simulink model "Assem1"  (R2015b)
settings: Solver=VariableStepAuto  StartTime=0.0  StopTime=10.0  RelTol=1e-3
undefined symbols (not defined in the file): Assem1, base, bearing, RootPart
libraries: mblibv1 x32
settings Model: Creator=kedar  LastModifiedBy=kedar
settings SimMechanicsCC: VisOnUpdateDiagram=on  VisDuringSimulation=on

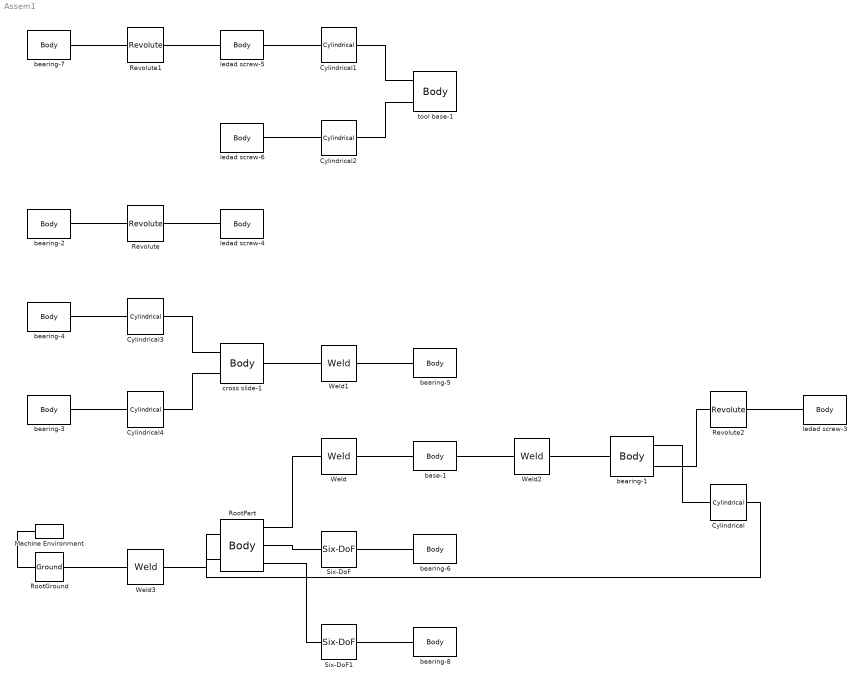
== system Assem1 ==
  Cylindrical : mblibv1/Joints/Cylindrical  LConnTagsString=__newl0  RConnTagsString=__newr0  UpdateFromCAD=on  PMImportedID=:-:Assem1/RootPart  NumSAPorts=0  CutJoint=off  MarkAsCut=off  Primitives=prismatic  PrimitiveProps=P1$WORLD$[-1,0,0]$prismatic#R1$WORLD$[1,0,0]$revolute  DialogClass=JointBlock  P1Axis=[-1,0,0]  R1Axis=[1,0,0]
  Cylindrical1 : mblibv1/Joints/Cylindrical  LConnTagsString=__newl0  RConnTagsString=__newr0  UpdateFromCAD=on  PMImportedID=ledad screw-5:-:tool base-1  NumSAPorts=0  CutJoint=off  MarkAsCut=off  Primitives=prismatic  PrimitiveProps=P1$WORLD$[0,0,-1]$prismatic#R1$WORLD$[0,0,-1]$revolute  DialogClass=JointBlock  P1Axis=[0,0,-1]  R1Axis=[0,0,-1]
  Cylindrical2 : mblibv1/Joints/Cylindrical  LConnTagsString=__newl0  RConnTagsString=__newr0  UpdateFromCAD=on  PMImportedID=ledad screw-6:-:tool base-1  NumSAPorts=0  CutJoint=off  MarkAsCut=off  Primitives=prismatic  PrimitiveProps=P1$WORLD$[0,0,-1]$prismatic#R1$WORLD$[0,0,1]$revolute  DialogClass=JointBlock  P1Axis=[0,0,-1]  R1Axis=[0,0,1]
  Cylindrical3 : mblibv1/Joints/Cylindrical  LConnTagsString=__newl0  RConnTagsString=__newr0  UpdateFromCAD=on  PMImportedID=bearing-4:-:cross slide-1  NumSAPorts=0  CutJoint=off  MarkAsCut=off  Primitives=prismatic  PrimitiveProps=P1$WORLD$[1,0,0]$prismatic#R1$WORLD$[-1,0,0]$revolute  DialogClass=JointBlock  P1Axis=[1,0,0]  R1Axis=[-1,0,0]
  Cylindrical4 : mblibv1/Joints/Cylindrical  LConnTagsString=__newl0  RConnTagsString=__newr0  UpdateFromCAD=on  PMImportedID=bearing-3:-:cross slide-1  NumSAPorts=0  CutJoint=off  MarkAsCut=off  Primitives=prismatic  PrimitiveProps=P1$WORLD$[1,0,0]$prismatic#R1$WORLD$[1,0,0]$revolute  DialogClass=JointBlock  P1Axis=[1,0,0]  R1Axis=[1,0,0]
  Machine Environment : mblibv1/Bodies/Machine Environment  PortType=env  PhysicalDomain=Mechanical  DialogTemplateClass=MECH.MachineEnvironment  SyncWhenCopied=off  Gravity=[0 -9.81 0]  GravityUnits=m/s^2  GravityAsSignal=off  Dimensionality=Auto-detect  AnalysisType=Forward dynamics  LinearAssemblyTolerance=1e-3  LinearAssemblyToleranceUnits=m  AngularAssemblyTolerance=1e-3  AngularAssemblyToleranceUnits=rad  ConstraintSolverType=Stabilizing  ConstraintRelTolerance=1e-4  ConstraintAbsTolerance=1e-4  UseRobustSingularityHandling=off  RedundancyAnalysisToleranceType=Automatically select tolerance  RedundancyAnalysisTolerance=1e-14  StatePerturbationType=Fixed  PerturbationSize=1e-5  VisualizeMachine=on  BodyVisualizationType=Use model default body geometries  BodyColorSelMode=Use model default  DefaultBodyColor=[1 0 0]
  Revolute : mblibv1/Joints/Revolute  LConnTagsString=__newl0  RConnTagsString=__newr0  UpdateFromCAD=on  PMImportedID=bearing-2:-:ledad screw-4  NumSAPorts=0  CutJoint=off  MarkAsCut=off  Primitives=prismatic  PrimitiveProps=R1$WORLD$[-1,0,0]$revolute  DialogClass=JointBlock  R1Axis=[-1,0,0]
  Revolute1 : mblibv1/Joints/Revolute  LConnTagsString=__newl0  RConnTagsString=__newr0  UpdateFromCAD=on  PMImportedID=bearing-7:-:ledad screw-5  NumSAPorts=0  CutJoint=off  MarkAsCut=off  Primitives=prismatic  PrimitiveProps=R1$WORLD$[0,0,1]$revolute  DialogClass=JointBlock  R1Axis=[0,0,1]
  Revolute2 : mblibv1/Joints/Revolute  LConnTagsString=__newl0  RConnTagsString=__newr0  UpdateFromCAD=on  PMImportedID=bearing-1:-:ledad screw-3  NumSAPorts=0  CutJoint=off  MarkAsCut=off  Primitives=prismatic  PrimitiveProps=R1$WORLD$[1,0,0]$revolute  DialogClass=JointBlock  R1Axis=[1,0,0]
  RootGround : mblibv1/Bodies/Ground  UpdateFromCAD=on  PMImportedID=RootGround  LeftPortType=env  RightPortType=workingframe  PhysicalDomain=Mechanical  DialogClass=GroundBlock  CoordPosition=[0.129768,0.219718,0.334095]  CoordPositionUnits=m  StateVectorMgrId=-1  MachineId=[0 0]  ShowEnvPort=on  ParameterChecksum=[0 0 0 0]  TopologyChecksum=[0 0 0 0]
  RootPart : mblibv1/Bodies/Body  LConnTagsString=CS3|CS4  RConnTagsString=CS2|CS5|CS6  UpdateFromCAD=on  PMImportedID=Assem1/RootPart  DialogClass=MechanicalBodyBlock  Mass=0  MassUnits=kg  InertiaUnits=kg*m^2  Inertia=[0,0,0;0,0,0;0,0,0]  Shape=Cylinder  ShapeDims=[1 1]  ShapeUnits=m  ShapeUse=false  Density=1  DensityUnits=kg/m^3  DensityUse=false  GraphicsMode=MACHINE_DEFAULT  BodyColorSelMode=MACHINE_DEFAULT  BodyColor=[1;0;0]  AttachedToCS=CS1  CG=Right$CG$[0.129768 0.219718 0.334095]$WORLD$WORLD$m$[1 0 0;0 1 0;0 0 1]$3x3 Transform$rad$WORLD$false$Assem1/RootPart::CG(AUTOGEN)  WorkingFrames=Right$CS1$[0 0 0]$WORLD$WORLD$m$[1 0 0;0 1 0;0 0 1]$3x3 Transform$rad$WORLD$false$Assem1/RootPart::CS1(AUTOGEN)#Right$CS2$[0.132232 0.182641 0.333778]$WORLD$WORLD$m$[1 0 0;0 1 0;0 0 1]$3x3 Transform$rad$WORLD$true$Assem1/RootPart:-:base-1::Assem1/RootPart(AUTOGEN)#Left$CS3$[0.312232 0.212641 0.513778]$WORLD$WORLD$m$[1 0 0;0 1 0;0 0 1]$3x3 Transform$rad$WORLD$true$:-:Assem1/RootPart::Assem1/RootPart(AUTOGEN)#Left$CS4$[0.129768 0.219718 0.334095]$WORLD$WORLD$m$[1 0 0;0 1 0;0 0 1]$3x3 Transform$rad$WORLD$true$Assem1/RootPart:-:RootGround::Assem1/RootPart(AUTOGEN)#Right$CS5$[0.129768 0.219718 0.334095]$WORLD$WORLD$m$[1 0 0;0 1 0;0 0 1]$3x3 Transform$rad$WORLD$true$Assem1/RootPart:-:bearing-6::Assem1/RootPart(AUTOGEN)#Right$CS6$[0.129768 0.219718 0.334095]$WORLD$WORLD$m$[1 0 0;0 1 0;0 0 1]$3x3 Transform$rad$WORLD$true$Assem1/RootPart:-:bearing-8::Assem1/RootPart(AUTOGEN)  CGPos=[0.129768 0.219718 0.334095]  CGRot=[1 0 0;0 1 0;0 0 1]  CS0Pos=[]  CS0Rot=[]  CS1Pos=[0 0 0]  CS1Rot=[1 0 0;0 1 0;0 0 1]  CS2Pos=[0.132232 0.182641 0.333778]  CS2Rot=[1 0 0;0 1 0;0 0 1]  CS3Pos=[0.312232 0.212641 0.513778]  CS3Rot=[1 0 0;0 1 0;0 0 1]  CS4Pos=[0.129768 0.219718 0.334095]  CS4Rot=[1 0 0;0 1 0;0 0 1]  CS5Pos=[0.129768 0.219718 0.334095]  CS5Rot=[1 0 0;0 1 0;0 0 1]  CS6Pos=[0.129768 0.219718 0.334095]  CS6Rot=[1 0 0;0 1 0;0 0 1]  CS7Pos=[]  CS7Rot=[]  CS8Pos=[]  CS8Rot=[]  CS9Pos=[]  CS9Rot=[]  CS10Pos=[]  CS10Rot=[]  CS11Pos=[]  CS11Rot=[]  CS12Pos=[]  CS12Rot=[]  CS13Pos=[]  CS13Rot=[]  CS14Pos=[]  CS14Rot=[]  CS15Pos=[]  CS15Rot=[]  CS16Pos=[]  CS16Rot=[]  CS17Pos=[]  CS17Rot=[]  CS18Pos=[]  CS18Rot=[]  CS19Pos=[]  CS19Rot=[]  CS20Pos=[]  CS20Rot=[]
  Six-DoF : mblibv1/Joints/Six-DoF  LConnTagsString=__newl0  RConnTagsString=__newr0  UpdateFromCAD=on  PMImportedID=Assem1/RootPart:-:bearing-6  NumSAPorts=0  CutJoint=off  MarkAsCut=off  Primitives=prismatic_prismatic  PrimitiveProps=P1$WORLD$[1,0,0]$prismatic#P2$WORLD$[0,1,0]$prismatic#P3$WORLD$[0,0,1]$prismatic#S$WORLD$[0,0,0]$spherical  DialogClass=JointBlock  P1Axis=[1,0,0]  P2Axis=[0,1,0]  P3Axis=[0,0,1]  SAxis=[0,0,0]
  Six-DoF1 : mblibv1/Joints/Six-DoF  LConnTagsString=__newl0  RConnTagsString=__newr0  UpdateFromCAD=on  PMImportedID=Assem1/RootPart:-:bearing-8  NumSAPorts=0  CutJoint=off  MarkAsCut=off  Primitives=prismatic_prismatic  PrimitiveProps=P1$WORLD$[1,0,0]$prismatic#P2$WORLD$[0,1,0]$prismatic#P3$WORLD$[0,0,1]$prismatic#S$WORLD$[0,0,0]$spherical  DialogClass=JointBlock  P1Axis=[1,0,0]  P2Axis=[0,1,0]  P3Axis=[0,0,1]  SAxis=[0,0,0]
  Weld : mblibv1/Joints/Weld  LConnTagsString=__newl0  RConnTagsString=__newr0  UpdateFromCAD=on  PMImportedID=Assem1/RootPart:-:base-1  NumSAPorts=0  CutJoint=off  MarkAsCut=off  Primitives=weld  PrimitiveProps=W$WORLD$[0.57735,0.57735,0.57735]$weld  DialogClass=JointBlock  WAxis=[0.57735,0.57735,0.57735]
  Weld1 : mblibv1/Joints/Weld  LConnTagsString=__newl0  RConnTagsString=__newr0  UpdateFromCAD=on  PMImportedID=bearing-5:-:cross slide-1  NumSAPorts=0  CutJoint=off  MarkAsCut=off  Primitives=weld  PrimitiveProps=W$WORLD$[0.57735,0.57735,0.57735]$weld  DialogClass=JointBlock  WAxis=[0.57735,0.57735,0.57735]
  Weld2 : mblibv1/Joints/Weld  LConnTagsString=__newl0  RConnTagsString=__newr0  UpdateFromCAD=on  PMImportedID=base-1:-:bearing-1  NumSAPorts=0  CutJoint=off  MarkAsCut=off  Primitives=weld  PrimitiveProps=W$WORLD$[0.57735,0.57735,0.57735]$weld  DialogClass=JointBlock  WAxis=[0.57735,0.57735,0.57735]
  Weld3 : mblibv1/Joints/Weld  LConnTagsString=__newl0  RConnTagsString=__newr0  UpdateFromCAD=on  PMImportedID=Assem1/RootPart:-:RootGround  NumSAPorts=0  CutJoint=off  MarkAsCut=off  Primitives=weld  PrimitiveProps=W$WORLD$[0.57735,0.57735,0.57735]$weld  DialogClass=JointBlock  WAxis=[0.57735,0.57735,0.57735]
  base-1 : mblibv1/Bodies/Body  LConnTagsString=CS2  RConnTagsString=CS3  UpdateFromCAD=on  PMImportedID=base-1  DialogClass=MechanicalBodyBlock  Mass=3.2  MassUnits=kg  InertiaUnits=kg*m^2  Inertia=[0.0427733,0,0;0,0.0853333,0;0,0,0.0427733]  Shape=Cylinder  ShapeDims=[1 1]  ShapeUnits=m  ShapeUse=false  Density=1  DensityUnits=kg/m^3  DensityUse=false  GraphicsMode=GFXFILE  GraphicsFileName=Assem1 - base-1.STL  BodyColorSelMode=COLORPALETTE  BodyColor=[0.792157;0.819608;0.933333]  AttachedToCS=CS1  CG=Right$CG$[0.132232 0.182641 0.333778]$WORLD$WORLD$m$[1 0 0;0 1 0;0 0 1]$3x3 Transform$rad$WORLD$false$base-1::CG(AUTOGEN)  WorkingFrames=Right$CS1$[0.132232 0.172641 0.333778]$WORLD$WORLD$m$[1 0 0;0 1 0;0 0 1]$3x3 Transform$rad$WORLD$false$base-1::CS1(AUTOGEN)#Left$CS2$[0.132232 0.182641 0.333778]$WORLD$WORLD$m$[1 0 0;0 1 0;0 0 1]$3x3 Transform$rad$WORLD$true$Assem1/RootPart:-:base-1::base-1(AUTOGEN)#Right$CS3$[0.332232 0.192641 0.533778]$WORLD$WORLD$m$[1 0 0;0 1 0;0 0 1]$3x3 Transform$rad$WORLD$true$base-1:-:bearing-1::base-1(AUTOGEN)  CGPos=[0.132232 0.182641 0.333778]  CGRot=[1 0 0;0 1 0;0 0 1]  CS0Pos=[]  CS0Rot=[]  CS1Pos=[0.132232 0.172641 0.333778]  CS1Rot=[1 0 0;0 1 0;0 0 1]  CS2Pos=[0.132232 0.182641 0.333778]  CS2Rot=[1 0 0;0 1 0;0 0 1]  CS3Pos=[0.332232 0.192641 0.533778]  CS3Rot=[1 0 0;0 1 0;0 0 1]  CS4Pos=[]  CS4Rot=[]  CS5Pos=[]  CS5Rot=[]  CS6Pos=[]  CS6Rot=[]  CS7Pos=[]  CS7Rot=[]  CS8Pos=[]  CS8Rot=[]  CS9Pos=[]  CS9Rot=[]  CS10Pos=[]  CS10Rot=[]  CS11Pos=[]  CS11Rot=[]  CS12Pos=[]  CS12Rot=[]  CS13Pos=[]  CS13Rot=[]  CS14Pos=[]  CS14Rot=[]  CS15Pos=[]  CS15Rot=[]  CS16Pos=[]  CS16Rot=[]  CS17Pos=[]  CS17Rot=[]  CS18Pos=[]  CS18Rot=[]  CS19Pos=[]  CS19Rot=[]  CS20Pos=[]  CS20Rot=[]
  bearing-1 : mblibv1/Bodies/Body  LConnTagsString=CS3  RConnTagsString=CS2|CS4  UpdateFromCAD=on  PMImportedID=bearing-1  DialogClass=MechanicalBodyBlock  Mass=0.0240913  MassUnits=kg  InertiaUnits=kg*m^2  Inertia=[4.82084e-06,0,0;0,4.82084e-06,0;0,0,8.03559e-06]  Shape=Cylinder  ShapeDims=[1 1]  ShapeUnits=m  ShapeUse=false  Density=1  DensityUnits=kg/m^3  DensityUse=false  GraphicsMode=GFXFILE  GraphicsFileName=Assem1 - bearing-1.STL  BodyColorSelMode=COLORPALETTE  BodyColor=[0.792157;0.819608;0.933333]  AttachedToCS=CS1  CG=Right$CG$[0.322232 0.212641 0.513778]$WORLD$WORLD$m$[0 0 -1;0 -1 0;-1 0 0]$3x3 Transform$rad$WORLD$false$bearing-1::CG(AUTOGEN)  WorkingFrames=Right$CS1$[0.332232 0.212641 0.513778]$WORLD$WORLD$m$[0 0 -1;0 -1 0;-1 0 0]$3x3 Transform$rad$WORLD$false$bearing-1::CS1(AUTOGEN)#Right$CS2$[0.312232 0.212641 0.513778]$WORLD$WORLD$m$[1 0 0;0 1 0;0 0 1]$3x3 Transform$rad$WORLD$true$:-:Assem1/RootPart::bearing-1(AUTOGEN)#Left$CS3$[0.332232 0.192641 0.533778]$WORLD$WORLD$m$[1 0 0;0 1 0;0 0 1]$3x3 Transform$rad$WORLD$true$base-1:-:bearing-1::bearing-1(AUTOGEN)#Right$CS4$[0.312232 0.212641 0.513778]$WORLD$WORLD$m$[1 0 0;0 1 0;0 0 1]$3x3 Transform$rad$WORLD$true$bearing-1:-:ledad screw-3::bearing-1(AUTOGEN)  CGPos=[0.322232 0.212641 0.513778]  CGRot=[0 0 -1;0 -1 0;-1 0 0]  CS0Pos=[]  CS0Rot=[]  CS1Pos=[0.332232 0.212641 0.513778]  CS1Rot=[0 0 -1;0 -1 0;-1 0 0]  CS2Pos=[0.312232 0.212641 0.513778]  CS2Rot=[1 0 0;0 1 0;0 0 1]  CS3Pos=[0.332232 0.192641 0.533778]  CS3Rot=[1 0 0;0 1 0;0 0 1]  CS4Pos=[0.312232 0.212641 0.513778]  CS4Rot=[1 0 0;0 1 0;0 0 1]  CS5Pos=[]  CS5Rot=[]  CS6Pos=[]  CS6Rot=[]  CS7Pos=[]  CS7Rot=[]  CS8Pos=[]  CS8Rot=[]  CS9Pos=[]  CS9Rot=[]  CS10Pos=[]  CS10Rot=[]  CS11Pos=[]  CS11Rot=[]  CS12Pos=[]  CS12Rot=[]  CS13Pos=[]  CS13Rot=[]  CS14Pos=[]  CS14Rot=[]  CS15Pos=[]  CS15Rot=[]  CS16Pos=[]  CS16Rot=[]  CS17Pos=[]  CS17Rot=[]  CS18Pos=[]  CS18Rot=[]  CS19Pos=[]  CS19Rot=[]  CS20Pos=[]  CS20Rot=[]
  bearing-2 : mblibv1/Bodies/Body  RConnTagsString=CS2  UpdateFromCAD=on  PMImportedID=bearing-2  DialogClass=MechanicalBodyBlock  Mass=0.0240913  MassUnits=kg  InertiaUnits=kg*m^2  Inertia=[4.82084e-06,0,0;0,4.82084e-06,0;0,0,8.03559e-06]  Shape=Cylinder  ShapeDims=[1 1]  ShapeUnits=m  ShapeUse=false  Density=1  DensityUnits=kg/m^3  DensityUse=false  GraphicsMode=GFXFILE  GraphicsFileName=Assem1 - bearing-2.STL  BodyColorSelMode=COLORPALETTE  BodyColor=[0.792157;0.819608;0.933333]  AttachedToCS=CS1  CG=Right$CG$[0.322232 0.212641 0.153778]$WORLD$WORLD$m$[0 0 1;0 -1 0;1 0 0]$3x3 Transform$rad$WORLD$false$bearing-2::CG(AUTOGEN)  WorkingFrames=Right$CS1$[0.312232 0.212641 0.153778]$WORLD$WORLD$m$[0 0 1;0 -1 0;1 0 0]$3x3 Transform$rad$WORLD$false$bearing-2::CS1(AUTOGEN)#Right$CS2$[0.332232 0.212641 0.153778]$WORLD$WORLD$m$[1 0 0;0 1 0;0 0 1]$3x3 Transform$rad$WORLD$true$bearing-2:-:ledad screw-4::bearing-2(AUTOGEN)  CGPos=[0.322232 0.212641 0.153778]  CGRot=[0 0 1;0 -1 0;1 0 0]  CS0Pos=[]  CS0Rot=[]  CS1Pos=[0.312232 0.212641 0.153778]  CS1Rot=[0 0 1;0 -1 0;1 0 0]  CS2Pos=[0.332232 0.212641 0.153778]  CS2Rot=[1 0 0;0 1 0;0 0 1]  CS3Pos=[]  CS3Rot=[]  CS4Pos=[]  CS4Rot=[]  CS5Pos=[]  CS5Rot=[]  CS6Pos=[]  CS6Rot=[]  CS7Pos=[]  CS7Rot=[]  CS8Pos=[]  CS8Rot=[]  CS9Pos=[]  CS9Rot=[]  CS10Pos=[]  CS10Rot=[]  CS11Pos=[]  CS11Rot=[]  CS12Pos=[]  CS12Rot=[]  CS13Pos=[]  CS13Rot=[]  CS14Pos=[]  CS14Rot=[]  CS15Pos=[]  CS15Rot=[]  CS16Pos=[]  CS16Rot=[]  CS17Pos=[]  CS17Rot=[]  CS18Pos=[]  CS18Rot=[]  CS19Pos=[]  CS19Rot=[]  CS20Pos=[]  CS20Rot=[]
  bearing-3 : mblibv1/Bodies/Body  RConnTagsString=CS2  UpdateFromCAD=on  PMImportedID=bearing-3  DialogClass=MechanicalBodyBlock  Mass=0.0240913  MassUnits=kg  InertiaUnits=kg*m^2  Inertia=[4.82084e-06,0,0;0,4.82084e-06,0;0,0,8.03559e-06]  Shape=Cylinder  ShapeDims=[1 1]  ShapeUnits=m  ShapeUse=false  Density=1  DensityUnits=kg/m^3  DensityUse=false  GraphicsMode=GFXFILE  GraphicsFileName=Assem1 - bearing-3.STL  BodyColorSelMode=COLORPALETTE  BodyColor=[0.792157;0.819608;0.933333]  AttachedToCS=CS1  CG=Right$CG$[-0.0577677 0.212641 0.513778]$WORLD$WORLD$m$[0 0 -1;0 -1 0;-1 0 0]$3x3 Transform$rad$WORLD$false$bearing-3::CG(AUTOGEN)  WorkingFrames=Right$CS1$[-0.0477677 0.212641 0.513778]$WORLD$WORLD$m$[0 0 -1;0 -1 0;-1 0 0]$3x3 Transform$rad$WORLD$false$bearing-3::CS1(AUTOGEN)#Right$CS2$[-0.0677677 0.212641 0.513778]$WORLD$WORLD$m$[1 0 0;0 1 0;0 0 1]$3x3 Transform$rad$WORLD$true$bearing-3:-:cross slide-1::bearing-3(AUTOGEN)  CGPos=[-0.0577677 0.212641 0.513778]  CGRot=[0 0 -1;0 -1 0;-1 0 0]  CS0Pos=[]  CS0Rot=[]  CS1Pos=[-0.0477677 0.212641 0.513778]  CS1Rot=[0 0 -1;0 -1 0;-1 0 0]  CS2Pos=[-0.0677677 0.212641 0.513778]  CS2Rot=[1 0 0;0 1 0;0 0 1]  CS3Pos=[]  CS3Rot=[]  CS4Pos=[]  CS4Rot=[]  CS5Pos=[]  CS5Rot=[]  CS6Pos=[]  CS6Rot=[]  CS7Pos=[]  CS7Rot=[]  CS8Pos=[]  CS8Rot=[]  CS9Pos=[]  CS9Rot=[]  CS10Pos=[]  CS10Rot=[]  CS11Pos=[]  CS11Rot=[]  CS12Pos=[]  CS12Rot=[]  CS13Pos=[]  CS13Rot=[]  CS14Pos=[]  CS14Rot=[]  CS15Pos=[]  CS15Rot=[]  CS16Pos=[]  CS16Rot=[]  CS17Pos=[]  CS17Rot=[]  CS18Pos=[]  CS18Rot=[]  CS19Pos=[]  CS19Rot=[]  CS20Pos=[]  CS20Rot=[]
  bearing-4 : mblibv1/Bodies/Body  RConnTagsString=CS2  UpdateFromCAD=on  PMImportedID=bearing-4  DialogClass=MechanicalBodyBlock  Mass=0.0240913  MassUnits=kg  InertiaUnits=kg*m^2  Inertia=[4.82084e-06,0,0;0,4.82084e-06,0;0,0,8.03559e-06]  Shape=Cylinder  ShapeDims=[1 1]  ShapeUnits=m  ShapeUse=false  Density=1  DensityUnits=kg/m^3  DensityUse=false  GraphicsMode=GFXFILE  GraphicsFileName=Assem1 - bearing-4.STL  BodyColorSelMode=COLORPALETTE  BodyColor=[0.792157;0.819608;0.933333]  AttachedToCS=CS1  CG=Right$CG$[-0.0577677 0.212641 0.153778]$WORLD$WORLD$m$[0 0 1;0 -1 0;1 0 0]$3x3 Transform$rad$WORLD$false$bearing-4::CG(AUTOGEN)  WorkingFrames=Right$CS1$[-0.0677677 0.212641 0.153778]$WORLD$WORLD$m$[0 0 1;0 -1 0;1 0 0]$3x3 Transform$rad$WORLD$false$bearing-4::CS1(AUTOGEN)#Right$CS2$[-0.0477677 0.212641 0.153778]$WORLD$WORLD$m$[1 0 0;0 1 0;0 0 1]$3x3 Transform$rad$WORLD$true$bearing-4:-:cross slide-1::bearing-4(AUTOGEN)  CGPos=[-0.0577677 0.212641 0.153778]  CGRot=[0 0 1;0 -1 0;1 0 0]  CS0Pos=[]  CS0Rot=[]  CS1Pos=[-0.0677677 0.212641 0.153778]  CS1Rot=[0 0 1;0 -1 0;1 0 0]  CS2Pos=[-0.0477677 0.212641 0.153778]  CS2Rot=[1 0 0;0 1 0;0 0 1]  CS3Pos=[]  CS3Rot=[]  CS4Pos=[]  CS4Rot=[]  CS5Pos=[]  CS5Rot=[]  CS6Pos=[]  CS6Rot=[]  CS7Pos=[]  CS7Rot=[]  CS8Pos=[]  CS8Rot=[]  CS9Pos=[]  CS9Rot=[]  CS10Pos=[]  CS10Rot=[]  CS11Pos=[]  CS11Rot=[]  CS12Pos=[]  CS12Rot=[]  CS13Pos=[]  CS13Rot=[]  CS14Pos=[]  CS14Rot=[]  CS15Pos=[]  CS15Rot=[]  CS16Pos=[]  CS16Rot=[]  CS17Pos=[]  CS17Rot=[]  CS18Pos=[]  CS18Rot=[]  CS19Pos=[]  CS19Rot=[]  CS20Pos=[]  CS20Rot=[]
  bearing-5 : mblibv1/Bodies/Body  LConnTagsString=CS2  UpdateFromCAD=on  PMImportedID=bearing-5  DialogClass=MechanicalBodyBlock  Mass=0.0240913  MassUnits=kg  InertiaUnits=kg*m^2  Inertia=[4.82084e-06,0,0;0,4.82084e-06,0;0,0,8.03559e-06]  Shape=Cylinder  ShapeDims=[1 1]  ShapeUnits=m  ShapeUse=false  Density=1  DensityUnits=kg/m^3  DensityUse=false  GraphicsMode=GFXFILE  GraphicsFileName=Assem1 - bearing-5.STL  BodyColorSelMode=COLORPALETTE  BodyColor=[0.792157;0.819608;0.933333]  AttachedToCS=CS1  CG=Right$CG$[0.236818 0.272641 0.523778]$WORLD$WORLD$m$[1 0 0;0 1 0;0 0 1]$3x3 Transform$rad$WORLD$false$bearing-5::CG(AUTOGEN)  WorkingFrames=Right$CS1$[0.236818 0.272641 0.513778]$WORLD$WORLD$m$[1 0 0;0 1 0;0 0 1]$3x3 Transform$rad$WORLD$false$bearing-5::CS1(AUTOGEN)#Left$CS2$[0.256818 0.232641 0.133778]$WORLD$WORLD$m$[1 0 0;0 1 0;0 0 1]$3x3 Transform$rad$WORLD$true$bearing-5:-:cross slide-1::bearing-5(AUTOGEN)  CGPos=[0.236818 0.272641 0.523778]  CGRot=[1 0 0;0 1 0;0 0 1]  CS0Pos=[]  CS0Rot=[]  CS1Pos=[0.236818 0.272641 0.513778]  CS1Rot=[1 0 0;0 1 0;0 0 1]  CS2Pos=[0.256818 0.232641 0.133778]  CS2Rot=[1 0 0;0 1 0;0 0 1]  CS3Pos=[]  CS3Rot=[]  CS4Pos=[]  CS4Rot=[]  CS5Pos=[]  CS5Rot=[]  CS6Pos=[]  CS6Rot=[]  CS7Pos=[]  CS7Rot=[]  CS8Pos=[]  CS8Rot=[]  CS9Pos=[]  CS9Rot=[]  CS10Pos=[]  CS10Rot=[]  CS11Pos=[]  CS11Rot=[]  CS12Pos=[]  CS12Rot=[]  CS13Pos=[]  CS13Rot=[]  CS14Pos=[]  CS14Rot=[]  CS15Pos=[]  CS15Rot=[]  CS16Pos=[]  CS16Rot=[]  CS17Pos=[]  CS17Rot=[]  CS18Pos=[]  CS18Rot=[]  CS19Pos=[]  CS19Rot=[]  CS20Pos=[]  CS20Rot=[]
  bearing-6 : mblibv1/Bodies/Body  LConnTagsString=CS2  UpdateFromCAD=on  PMImportedID=bearing-6  DialogClass=MechanicalBodyBlock  Mass=0.0240913  MassUnits=kg  InertiaUnits=kg*m^2  Inertia=[4.82084e-06,0,0;0,4.82084e-06,0;0,0,8.03559e-06]  Shape=Cylinder  ShapeDims=[1 1]  ShapeUnits=m  ShapeUse=false  Density=1  DensityUnits=kg/m^3  DensityUse=false  GraphicsMode=GFXFILE  GraphicsFileName=Assem1 - bearing-6.STL  BodyColorSelMode=COLORPALETTE  BodyColor=[0.792157;0.819608;0.933333]  AttachedToCS=CS1  CG=Right$CG$[0.236818 0.272641 0.143778]$WORLD$WORLD$m$[1 0 0;0 1 0;0 0 1]$3x3 Transform$rad$WORLD$false$bearing-6::CG(AUTOGEN)  WorkingFrames=Right$CS1$[0.236818 0.272641 0.133778]$WORLD$WORLD$m$[1 0 0;0 1 0;0 0 1]$3x3 Transform$rad$WORLD$false$bearing-6::CS1(AUTOGEN)#Left$CS2$[0.236818 0.272641 0.143778]$WORLD$WORLD$m$[1 0 0;0 1 0;0 0 1]$3x3 Transform$rad$WORLD$true$Assem1/RootPart:-:bearing-6::bearing-6(AUTOGEN)  CGPos=[0.236818 0.272641 0.143778]  CGRot=[1 0 0;0 1 0;0 0 1]  CS0Pos=[]  CS0Rot=[]  CS1Pos=[0.236818 0.272641 0.133778]  CS1Rot=[1 0 0;0 1 0;0 0 1]  CS2Pos=[0.236818 0.272641 0.143778]  CS2Rot=[1 0 0;0 1 0;0 0 1]  CS3Pos=[]  CS3Rot=[]  CS4Pos=[]  CS4Rot=[]  CS5Pos=[]  CS5Rot=[]  CS6Pos=[]  CS6Rot=[]  CS7Pos=[]  CS7Rot=[]  CS8Pos=[]  CS8Rot=[]  CS9Pos=[]  CS9Rot=[]  CS10Pos=[]  CS10Rot=[]  CS11Pos=[]  CS11Rot=[]  CS12Pos=[]  CS12Rot=[]  CS13Pos=[]  CS13Rot=[]  CS14Pos=[]  CS14Rot=[]  CS15Pos=[]  CS15Rot=[]  CS16Pos=[]  CS16Rot=[]  CS17Pos=[]  CS17Rot=[]  CS18Pos=[]  CS18Rot=[]  CS19Pos=[]  CS19Rot=[]  CS20Pos=[]  CS20Rot=[]
  bearing-7 : mblibv1/Bodies/Body  RConnTagsString=CS2  UpdateFromCAD=on  PMImportedID=bearing-7  DialogClass=MechanicalBodyBlock  Mass=0.0240913  MassUnits=kg  InertiaUnits=kg*m^2  Inertia=[4.82084e-06,0,0;0,4.82084e-06,0;0,0,8.03559e-06]  Shape=Cylinder  ShapeDims=[1 1]  ShapeUnits=m  ShapeUse=false  Density=1  DensityUnits=kg/m^3  DensityUse=false  GraphicsMode=GFXFILE  GraphicsFileName=Assem1 - bearing-7.STL  BodyColorSelMode=COLORPALETTE  BodyColor=[0.792157;0.819608;0.933333]  AttachedToCS=CS1  CG=Right$CG$[0.0268176 0.272641 0.523778]$WORLD$WORLD$m$[-1 0 0;0 1 0;0 0 -1]$3x3 Transform$rad$WORLD$false$bearing-7::CG(AUTOGEN)  WorkingFrames=Right$CS1$[0.0268176 0.272641 0.533778]$WORLD$WORLD$m$[-1 0 0;0 1 0;0 0 -1]$3x3 Transform$rad$WORLD$false$bearing-7::CS1(AUTOGEN)#Right$CS2$[0.0268176 0.272641 0.513778]$WORLD$WORLD$m$[1 0 0;0 1 0;0 0 1]$3x3 Transform$rad$WORLD$true$bearing-7:-:ledad screw-5::bearing-7(AUTOGEN)  CGPos=[0.0268176 0.272641 0.523778]  CGRot=[-1 0 0;0 1 0;0 0 -1]  CS0Pos=[]  CS0Rot=[]  CS1Pos=[0.0268176 0.272641 0.533778]  CS1Rot=[-1 0 0;0 1 0;0 0 -1]  CS2Pos=[0.0268176 0.272641 0.513778]  CS2Rot=[1 0 0;0 1 0;0 0 1]  CS3Pos=[]  CS3Rot=[]  CS4Pos=[]  CS4Rot=[]  CS5Pos=[]  CS5Rot=[]  CS6Pos=[]  CS6Rot=[]  CS7Pos=[]  CS7Rot=[]  CS8Pos=[]  CS8Rot=[]  CS9Pos=[]  CS9Rot=[]  CS10Pos=[]  CS10Rot=[]  CS11Pos=[]  CS11Rot=[]  CS12Pos=[]  CS12Rot=[]  CS13Pos=[]  CS13Rot=[]  CS14Pos=[]  CS14Rot=[]  CS15Pos=[]  CS15Rot=[]  CS16Pos=[]  CS16Rot=[]  CS17Pos=[]  CS17Rot=[]  CS18Pos=[]  CS18Rot=[]  CS19Pos=[]  CS19Rot=[]  CS20Pos=[]  CS20Rot=[]
  bearing-8 : mblibv1/Bodies/Body  LConnTagsString=CS2  UpdateFromCAD=on  PMImportedID=bearing-8  DialogClass=MechanicalBodyBlock  Mass=0.0240913  MassUnits=kg  InertiaUnits=kg*m^2  Inertia=[4.82084e-06,0,0;0,4.82084e-06,0;0,0,8.03559e-06]  Shape=Cylinder  ShapeDims=[1 1]  ShapeUnits=m  ShapeUse=false  Density=1  DensityUnits=kg/m^3  DensityUse=false  GraphicsMode=GFXFILE  GraphicsFileName=Assem1 - bearing-8.STL  BodyColorSelMode=COLORPALETTE  BodyColor=[0.792157;0.819608;0.933333]  AttachedToCS=CS1  CG=Right$CG$[0.0268176 0.272641 0.143778]$WORLD$WORLD$m$[-1 0 0;0 1 0;0 0 -1]$3x3 Transform$rad$WORLD$false$bearing-8::CG(AUTOGEN)  WorkingFrames=Right$CS1$[0.0268176 0.272641 0.153778]$WORLD$WORLD$m$[-1 0 0;0 1 0;0 0 -1]$3x3 Transform$rad$WORLD$false$bearing-8::CS1(AUTOGEN)#Left$CS2$[0.0268176 0.272641 0.143778]$WORLD$WORLD$m$[1 0 0;0 1 0;0 0 1]$3x3 Transform$rad$WORLD$true$Assem1/RootPart:-:bearing-8::bearing-8(AUTOGEN)  CGPos=[0.0268176 0.272641 0.143778]  CGRot=[-1 0 0;0 1 0;0 0 -1]  CS0Pos=[]  CS0Rot=[]  CS1Pos=[0.0268176 0.272641 0.153778]  CS1Rot=[-1 0 0;0 1 0;0 0 -1]  CS2Pos=[0.0268176 0.272641 0.143778]  CS2Rot=[1 0 0;0 1 0;0 0 1]  CS3Pos=[]  CS3Rot=[]  CS4Pos=[]  CS4Rot=[]  CS5Pos=[]  CS5Rot=[]  CS6Pos=[]  CS6Rot=[]  CS7Pos=[]  CS7Rot=[]  CS8Pos=[]  CS8Rot=[]  CS9Pos=[]  CS9Rot=[]  CS10Pos=[]  CS10Rot=[]  CS11Pos=[]  CS11Rot=[]  CS12Pos=[]  CS12Rot=[]  CS13Pos=[]  CS13Rot=[]  CS14Pos=[]  CS14Rot=[]  CS15Pos=[]  CS15Rot=[]  CS16Pos=[]  CS16Rot=[]  CS17Pos=[]  CS17Rot=[]  CS18Pos=[]  CS18Rot=[]  CS19Pos=[]  CS19Rot=[]  CS20Pos=[]  CS20Rot=[]
  cross slide-1 : mblibv1/Bodies/Body  LConnTagsString=CS3|CS4  RConnTagsString=CS2  UpdateFromCAD=on  PMImportedID=cross slide-1  DialogClass=MechanicalBodyBlock  Mass=2.1543  MassUnits=kg  InertiaUnits=kg*m^2  Inertia=[0.0125155,0,0;0,0.043986,0;0,0,0.0319109]  Shape=Cylinder  ShapeDims=[1 1]  ShapeUnits=m  ShapeUse=false  Density=1  DensityUnits=kg/m^3  DensityUse=false  GraphicsMode=GFXFILE  GraphicsFileName=Assem1 - cross slide-1.STL  BodyColorSelMode=COLORPALETTE  BodyColor=[0.792157;0.819608;0.933333]  AttachedToCS=CS1  CG=Right$CG$[0.131818 0.240492 0.333778]$WORLD$WORLD$m$[0 0 1;0 -1 0;1 0 0]$3x3 Transform$rad$WORLD$false$cross slide-1::CG(AUTOGEN)  WorkingFrames=Right$CS1$[0.131818 0.252641 0.333778]$WORLD$WORLD$m$[0 0 1;0 -1 0;1 0 0]$3x3 Transform$rad$WORLD$false$cross slide-1::CS1(AUTOGEN)#Right$CS2$[0.256818 0.232641 0.133778]$WORLD$WORLD$m$[1 0 0;0 1 0;0 0 1]$3x3 Transform$rad$WORLD$true$bearing-5:-:cross slide-1::cross slide-1(AUTOGEN)#Left$CS3$[-0.0477677 0.212641 0.153778]$WORLD$WORLD$m$[1 0 0;0 1 0;0 0 1]$3x3 Transform$rad$WORLD$true$bearing-4:-:cross slide-1::cross slide-1(AUTOGEN)#Left$CS4$[-0.0677677 0.212641 0.513778]$WORLD$WORLD$m$[1 0 0;0 1 0;0 0 1]$3x3 Transform$rad$WORLD$true$bearing-3:-:cross slide-1::cross slide-1(AUTOGEN)  CGPos=[0.131818 0.240492 0.333778]  CGRot=[0 0 1;0 -1 0;1 0 0]  CS0Pos=[]  CS0Rot=[]  CS1Pos=[0.131818 0.252641 0.333778]  CS1Rot=[0 0 1;0 -1 0;1 0 0]  CS2Pos=[0.256818 0.232641 0.133778]  CS2Rot=[1 0 0;0 1 0;0 0 1]  CS3Pos=[-0.0477677 0.212641 0.153778]  CS3Rot=[1 0 0;0 1 0;0 0 1]  CS4Pos=[-0.0677677 0.212641 0.513778]  CS4Rot=[1 0 0;0 1 0;0 0 1]  CS5Pos=[]  CS5Rot=[]  CS6Pos=[]  CS6Rot=[]  CS7Pos=[]  CS7Rot=[]  CS8Pos=[]  CS8Rot=[]  CS9Pos=[]  CS9Rot=[]  CS10Pos=[]  CS10Rot=[]  CS11Pos=[]  CS11Rot=[]  CS12Pos=[]  CS12Rot=[]  CS13Pos=[]  CS13Rot=[]  CS14Pos=[]  CS14Rot=[]  CS15Pos=[]  CS15Rot=[]  CS16Pos=[]  CS16Rot=[]  CS17Pos=[]  CS17Rot=[]  CS18Pos=[]  CS18Rot=[]  CS19Pos=[]  CS19Rot=[]  CS20Pos=[]  CS20Rot=[]
  ledad screw-3 : mblibv1/Bodies/Body  LConnTagsString=CS2  UpdateFromCAD=on  PMImportedID=ledad screw-3  DialogClass=MechanicalBodyBlock  Mass=0.15708  MassUnits=kg  InertiaUnits=kg*m^2  Inertia=[0.00327642,0,0;0,0.00327642,0;0,0,7.85398e-06]  Shape=Cylinder  ShapeDims=[1 1]  ShapeUnits=m  ShapeUse=false  Density=1  DensityUnits=kg/m^3  DensityUse=false  GraphicsMode=GFXFILE  GraphicsFileName=Assem1 - ledad screw-3.STL  BodyColorSelMode=COLORPALETTE  BodyColor=[0.792157;0.819608;0.933333]  AttachedToCS=CS1  CG=Right$CG$[0.0822323 0.212641 0.513778]$WORLD$WORLD$m$[0 0 1;0 1 0;-1 0 0]$3x3 Transform$rad$WORLD$false$ledad screw-3::CG(AUTOGEN)  WorkingFrames=Right$CS1$[-0.167768 0.212641 0.513778]$WORLD$WORLD$m$[0 0 1;0 1 0;-1 0 0]$3x3 Transform$rad$WORLD$false$ledad screw-3::CS1(AUTOGEN)#Left$CS2$[0.312232 0.212641 0.513778]$WORLD$WORLD$m$[1 0 0;0 1 0;0 0 1]$3x3 Transform$rad$WORLD$true$bearing-1:-:ledad screw-3::ledad screw-3(AUTOGEN)  CGPos=[0.0822323 0.212641 0.513778]  CGRot=[0 0 1;0 1 0;-1 0 0]  CS0Pos=[]  CS0Rot=[]  CS1Pos=[-0.167768 0.212641 0.513778]  CS1Rot=[0 0 1;0 1 0;-1 0 0]  CS2Pos=[0.312232 0.212641 0.513778]  CS2Rot=[1 0 0;0 1 0;0 0 1]  CS3Pos=[]  CS3Rot=[]  CS4Pos=[]  CS4Rot=[]  CS5Pos=[]  CS5Rot=[]  CS6Pos=[]  CS6Rot=[]  CS7Pos=[]  CS7Rot=[]  CS8Pos=[]  CS8Rot=[]  CS9Pos=[]  CS9Rot=[]  CS10Pos=[]  CS10Rot=[]  CS11Pos=[]  CS11Rot=[]  CS12Pos=[]  CS12Rot=[]  CS13Pos=[]  CS13Rot=[]  CS14Pos=[]  CS14Rot=[]  CS15Pos=[]  CS15Rot=[]  CS16Pos=[]  CS16Rot=[]  CS17Pos=[]  CS17Rot=[]  CS18Pos=[]  CS18Rot=[]  CS19Pos=[]  CS19Rot=[]  CS20Pos=[]  CS20Rot=[]
  ledad screw-4 : mblibv1/Bodies/Body  LConnTagsString=CS2  UpdateFromCAD=on  PMImportedID=ledad screw-4  DialogClass=MechanicalBodyBlock  Mass=0.15708  MassUnits=kg  InertiaUnits=kg*m^2  Inertia=[0.00327642,0,0;0,0.00327642,0;0,0,7.85398e-06]  Shape=Cylinder  ShapeDims=[1 1]  ShapeUnits=m  ShapeUse=false  Density=1  DensityUnits=kg/m^3  DensityUse=false  GraphicsMode=GFXFILE  GraphicsFileName=Assem1 - ledad screw-4.STL  BodyColorSelMode=COLORPALETTE  BodyColor=[0.792157;0.819608;0.933333]  AttachedToCS=CS1  CG=Right$CG$[0.0822323 0.212641 0.153778]$WORLD$WORLD$m$[0 0 -1;0 1 0;1 0 0]$3x3 Transform$rad$WORLD$false$ledad screw-4::CG(AUTOGEN)  WorkingFrames=Right$CS1$[0.332232 0.212641 0.153778]$WORLD$WORLD$m$[0 0 -1;0 1 0;1 0 0]$3x3 Transform$rad$WORLD$false$ledad screw-4::CS1(AUTOGEN)#Left$CS2$[0.332232 0.212641 0.153778]$WORLD$WORLD$m$[1 0 0;0 1 0;0 0 1]$3x3 Transform$rad$WORLD$true$bearing-2:-:ledad screw-4::ledad screw-4(AUTOGEN)  CGPos=[0.0822323 0.212641 0.153778]  CGRot=[0 0 -1;0 1 0;1 0 0]  CS0Pos=[]  CS0Rot=[]  CS1Pos=[0.332232 0.212641 0.153778]  CS1Rot=[0 0 -1;0 1 0;1 0 0]  CS2Pos=[0.332232 0.212641 0.153778]  CS2Rot=[1 0 0;0 1 0;0 0 1]  CS3Pos=[]  CS3Rot=[]  CS4Pos=[]  CS4Rot=[]  CS5Pos=[]  CS5Rot=[]  CS6Pos=[]  CS6Rot=[]  CS7Pos=[]  CS7Rot=[]  CS8Pos=[]  CS8Rot=[]  CS9Pos=[]  CS9Rot=[]  CS10Pos=[]  CS10Rot=[]  CS11Pos=[]  CS11Rot=[]  CS12Pos=[]  CS12Rot=[]  CS13Pos=[]  CS13Rot=[]  CS14Pos=[]  CS14Rot=[]  CS15Pos=[]  CS15Rot=[]  CS16Pos=[]  CS16Rot=[]  CS17Pos=[]  CS17Rot=[]  CS18Pos=[]  CS18Rot=[]  CS19Pos=[]  CS19Rot=[]  CS20Pos=[]  CS20Rot=[]
  ledad screw-5 : mblibv1/Bodies/Body  LConnTagsString=CS3  RConnTagsString=CS2  UpdateFromCAD=on  PMImportedID=ledad screw-5  DialogClass=MechanicalBodyBlock  Mass=0.15708  MassUnits=kg  InertiaUnits=kg*m^2  Inertia=[0.00327642,0,0;0,0.00327642,0;0,0,7.85398e-06]  Shape=Cylinder  ShapeDims=[1 1]  ShapeUnits=m  ShapeUse=false  Density=1  DensityUnits=kg/m^3  DensityUse=false  GraphicsMode=GFXFILE  GraphicsFileName=Assem1 - ledad screw-5.STL  BodyColorSelMode=COLORPALETTE  BodyColor=[0.792157;0.819608;0.933333]  AttachedToCS=CS1  CG=Right$CG$[0.0268176 0.272641 0.283778]$WORLD$WORLD$m$[0.999997 -0.00229785 0;0.00229785 0.999997 0;0 0 1]$3x3 Transform$rad$WORLD$false$ledad screw-5::CG(AUTOGEN)  WorkingFrames=Right$CS1$[0.0268176 0.272641 0.0337781]$WORLD$WORLD$m$[0.999997 -0.00229785 0;0.00229785 0.999997 0;0 0 1]$3x3 Transform$rad$WORLD$false$ledad screw-5::CS1(AUTOGEN)#Right$CS2$[0.0268176 0.272641 0.533778]$WORLD$WORLD$m$[1 0 0;0 1 0;0 0 1]$3x3 Transform$rad$WORLD$true$ledad screw-5:-:tool base-1::ledad screw-5(AUTOGEN)#Left$CS3$[0.0268176 0.272641 0.513778]$WORLD$WORLD$m$[1 0 0;0 1 0;0 0 1]$3x3 Transform$rad$WORLD$true$bearing-7:-:ledad screw-5::ledad screw-5(AUTOGEN)  CGPos=[0.0268176 0.272641 0.283778]  CGRot=[0.999997 -0.00229785 0;0.00229785 0.999997 0;0 0 1]  CS0Pos=[]  CS0Rot=[]  CS1Pos=[0.0268176 0.272641 0.0337781]  CS1Rot=[0.999997 -0.00229785 0;0.00229785 0.999997 0;0 0 1]  CS2Pos=[0.0268176 0.272641 0.533778]  CS2Rot=[1 0 0;0 1 0;0 0 1]  CS3Pos=[0.0268176 0.272641 0.513778]  CS3Rot=[1 0 0;0 1 0;0 0 1]  CS4Pos=[]  CS4Rot=[]  CS5Pos=[]  CS5Rot=[]  CS6Pos=[]  CS6Rot=[]  CS7Pos=[]  CS7Rot=[]  CS8Pos=[]  CS8Rot=[]  CS9Pos=[]  CS9Rot=[]  CS10Pos=[]  CS10Rot=[]  CS11Pos=[]  CS11Rot=[]  CS12Pos=[]  CS12Rot=[]  CS13Pos=[]  CS13Rot=[]  CS14Pos=[]  CS14Rot=[]  CS15Pos=[]  CS15Rot=[]  CS16Pos=[]  CS16Rot=[]  CS17Pos=[]  CS17Rot=[]  CS18Pos=[]  CS18Rot=[]  CS19Pos=[]  CS19Rot=[]  CS20Pos=[]  CS20Rot=[]
  ledad screw-6 : mblibv1/Bodies/Body  RConnTagsString=CS2  UpdateFromCAD=on  PMImportedID=ledad screw-6  DialogClass=MechanicalBodyBlock  Mass=0.15708  MassUnits=kg  InertiaUnits=kg*m^2  Inertia=[0.00327642,0,0;0,0.00327642,0;0,0,7.85398e-06]  Shape=Cylinder  ShapeDims=[1 1]  ShapeUnits=m  ShapeUse=false  Density=1  DensityUnits=kg/m^3  DensityUse=false  GraphicsMode=GFXFILE  GraphicsFileName=Assem1 - ledad screw-6.STL  BodyColorSelMode=COLORPALETTE  BodyColor=[0.792157;0.819608;0.933333]  AttachedToCS=CS1  CG=Right$CG$[0.236818 0.272641 0.283778]$WORLD$WORLD$m$[-0.999997 0.00229785 0;0.00229785 0.999997 0;0 0 -1]$3x3 Transform$rad$WORLD$false$ledad screw-6::CG(AUTOGEN)  WorkingFrames=Right$CS1$[0.236818 0.272641 0.533778]$WORLD$WORLD$m$[-0.999997 0.00229785 0;0.00229785 0.999997 0;0 0 -1]$3x3 Transform$rad$WORLD$false$ledad screw-6::CS1(AUTOGEN)#Right$CS2$[0.236818 0.272641 0.0337781]$WORLD$WORLD$m$[1 0 0;0 1 0;0 0 1]$3x3 Transform$rad$WORLD$true$ledad screw-6:-:tool base-1::ledad screw-6(AUTOGEN)  CGPos=[0.236818 0.272641 0.283778]  CGRot=[-0.999997 0.00229785 0;0.00229785 0.999997 0;0 0 -1]  CS0Pos=[]  CS0Rot=[]  CS1Pos=[0.236818 0.272641 0.533778]  CS1Rot=[-0.999997 0.00229785 0;0.00229785 0.999997 0;0 0 -1]  CS2Pos=[0.236818 0.272641 0.0337781]  CS2Rot=[1 0 0;0 1 0;0 0 1]  CS3Pos=[]  CS3Rot=[]  CS4Pos=[]  CS4Rot=[]  CS5Pos=[]  CS5Rot=[]  CS6Pos=[]  CS6Rot=[]  CS7Pos=[]  CS7Rot=[]  CS8Pos=[]  CS8Rot=[]  CS9Pos=[]  CS9Rot=[]  CS10Pos=[]  CS10Rot=[]  CS11Pos=[]  CS11Rot=[]  CS12Pos=[]  CS12Rot=[]  CS13Pos=[]  CS13Rot=[]  CS14Pos=[]  CS14Rot=[]  CS15Pos=[]  CS15Rot=[]  CS16Pos=[]  CS16Rot=[]  CS17Pos=[]  CS17Rot=[]  CS18Pos=[]  CS18Rot=[]  CS19Pos=[]  CS19Rot=[]  CS20Pos=[]  CS20Rot=[]
  tool base-1 : mblibv1/Bodies/Body  LConnTagsString=CS2|CS3  UpdateFromCAD=on  PMImportedID=tool base-1  DialogClass=MechanicalBodyBlock  Mass=0.757168  MassUnits=kg  InertiaUnits=kg*m^2  Inertia=[0.000841576,0,0;0,0.00611151,0;0,0,0.00569114]  Shape=Cylinder  ShapeDims=[1 1]  ShapeUnits=m  ShapeUse=false  Density=1  DensityUnits=kg/m^3  DensityUse=false  GraphicsMode=GFXFILE  GraphicsFileName=Assem1 - tool base-1.STL  BodyColorSelMode=COLORPALETTE  BodyColor=[0.792157;0.819608;0.933333]  AttachedToCS=CS1  CG=Right$CG$[0.131818 0.292452 0.357429]$WORLD$WORLD$m$[1 0 0;0 -1 0;0 0 -1]$3x3 Transform$rad$WORLD$false$tool base-1::CG(AUTOGEN)  WorkingFrames=Right$CS1$[0.131818 0.312641 0.407429]$WORLD$WORLD$m$[1 0 0;0 -1 0;0 0 -1]$3x3 Transform$rad$WORLD$false$tool base-1::CS1(AUTOGEN)#Left$CS2$[0.0268176 0.272641 0.533778]$WORLD$WORLD$m$[1 0 0;0 1 0;0 0 1]$3x3 Transform$rad$WORLD$true$ledad screw-5:-:tool base-1::tool base-1(AUTOGEN)#Left$CS3$[0.236818 0.272641 0.0337781]$WORLD$WORLD$m$[1 0 0;0 1 0;0 0 1]$3x3 Transform$rad$WORLD$true$ledad screw-6:-:tool base-1::tool base-1(AUTOGEN)  CGPos=[0.131818 0.292452 0.357429]  CGRot=[1 0 0;0 -1 0;0 0 -1]  CS0Pos=[]  CS0Rot=[]  CS1Pos=[0.131818 0.312641 0.407429]  CS1Rot=[1 0 0;0 -1 0;0 0 -1]  CS2Pos=[0.0268176 0.272641 0.533778]  CS2Rot=[1 0 0;0 1 0;0 0 1]  CS3Pos=[0.236818 0.272641 0.0337781]  CS3Rot=[1 0 0;0 1 0;0 0 1]  CS4Pos=[]  CS4Rot=[]  CS5Pos=[]  CS5Rot=[]  CS6Pos=[]  CS6Rot=[]  CS7Pos=[]  CS7Rot=[]  CS8Pos=[]  CS8Rot=[]  CS9Pos=[]  CS9Rot=[]  CS10Pos=[]  CS10Rot=[]  CS11Pos=[]  CS11Rot=[]  CS12Pos=[]  CS12Rot=[]  CS13Pos=[]  CS13Rot=[]  CS14Pos=[]  CS14Rot=[]  CS15Pos=[]  CS15Rot=[]  CS16Pos=[]  CS16Rot=[]  CS17Pos=[]  CS17Rot=[]  CS18Pos=[]  CS18Rot=[]  CS19Pos=[]  CS19Rot=[]  CS20Pos=[]  CS20Rot=[]
  connections:
  RootPart/RConn1 -- Weld/LConn1
  Weld/RConn1 -- base-1/LConn1
  bearing-1/RConn1 -- Cylindrical/LConn1
  Cylindrical/RConn1 -- RootPart/LConn1
  ledad screw-5/RConn1 -- Cylindrical1/LConn1
  Cylindrical1/RConn1 -- tool base-1/LConn1
  ledad screw-6/RConn1 -- Cylindrical2/LConn1
  Cylindrical2/RConn1 -- tool base-1/LConn2
  bearing-2/RConn1 -- Revolute/LConn1
  Revolute/RConn1 -- ledad screw-4/LConn1
  cross slide-1/RConn1 -- Weld1/LConn1
  Weld1/RConn1 -- bearing-5/LConn1
  bearing-4/RConn1 -- Cylindrical3/LConn1
  Cylindrical3/RConn1 -- cross slide-1/LConn1
  bearing-3/RConn1 -- Cylindrical4/LConn1
  Cylindrical4/RConn1 -- cross slide-1/LConn2
  bearing-7/RConn1 -- Revolute1/LConn1
  Revolute1/RConn1 -- ledad screw-5/LConn1
  base-1/RConn1 -- Weld2/LConn1
  Weld2/RConn1 -- bearing-1/LConn1
  bearing-1/RConn2 -- Revolute2/LConn1
  Revolute2/RConn1 -- ledad screw-3/LConn1
  RootGround/RConn1 -- Weld3/LConn1
  Weld3/RConn1 -- RootPart/LConn2
  RootPart/RConn2 -- Six-DoF/LConn1
  Six-DoF/RConn1 -- bearing-6/LConn1
  RootPart/RConn3 -- Six-DoF1/LConn1
  Six-DoF1/RConn1 -- bearing-8/LConn1
  RootGround/LConn1 -- Machine Environment/RConn1
